simulink model "non_linear_cartesian_controller"  (R2024b)
settings: Solver=VariableStepAuto  StartTime=0.0  StopTime=40  RelTol=1e-3
undefined symbols (not defined in the file or in its folder): extractTop2x2, non_linear_m, non_linear_vcfg
libraries: roblocks x6

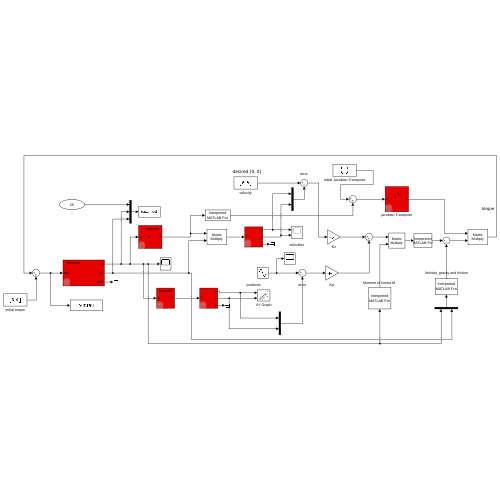
[thumbnail: Simulink's stored preview of the top-level diagram]
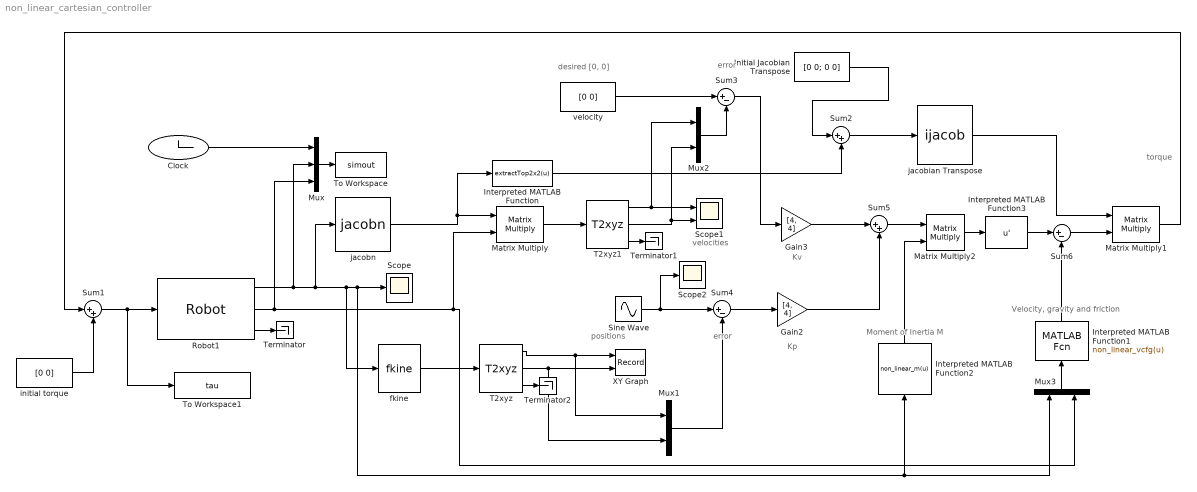
== system non_linear_cartesian_controller ==
  note: Kp
  note: Kv
  note: Moment of Inertia M
  note: error
  note: error
  note: velocities
  note: desired [0, 0]
  note: positions
  note: torque
  note: Velocity, gravity and friction
  Clock : Clock
  Gain2 : Gain  Gain=[4, 4]
  Gain3 : Gain  Gain=[4, 4]
  Initial Jacobian Transpose : Constant  Value=[0 0; 0 0]
  Interpreted MATLAB Function : MATLABFcn  MATLABFcn=extractTop2x2(u)  OutputDimensions=[2 2]  Output1D=off
  Interpreted MATLAB Function1 : MATLABFcn  MATLABFcn=non_linear_vcfg(u)  OutputDimensions=[2 1]  Output1D=off
  Interpreted MATLAB Function2 : MATLABFcn  MATLABFcn=non_linear_m(u)  OutputDimensions=[2 2]  Output1D=off
  Interpreted MATLAB Function3 : MATLABFcn  MATLABFcn=u'  OutputDimensions=[2 1]  Output1D=off
  Matrix Multiply : Product  Multiplication=Matrix(*)
  Matrix Multiply1 : Product  Multiplication=Matrix(*)
  Matrix Multiply2 : Product  Multiplication=Matrix(*)
  Mux : Mux  Inputs=3
  Mux1 : Mux  Inputs=2
  Mux2 : Mux  Inputs=2
  Mux3 : Mux  Inputs=2
  Robot1 : roblocks/Robot  robot=robot  q0=[0 0 0 0 0 0]
      link override Integrator: InitialCondition=[1 1]
      link override Integrator1: InitialCondition=[1 1]
  Scope : Scope
  Scope1 : Scope  NumInputPorts=2
  Scope2 : Scope
  Sine Wave : Sin  Amplitude=0.5  Bias=1  Frequency=1.256  SampleTime=0
  Sum1 : Sum  Inputs=|++
  Sum2 : Sum  Inputs=|++
  Sum3 : Sum  Inputs=|+-
  Sum4 : Sum  Inputs=|+-
  Sum5 : Sum  Inputs=|++
  Sum6 : Sum  Inputs=|+-
  T2xyz : roblocks/T2xyz
  T2xyz1 : roblocks/T2xyz
      link override MATLAB Fcn: MATLABFcn=transljac(u)
  Terminator : Terminator
  Terminator1 : Terminator
  Terminator2 : Terminator
  To Workspace : ToWorkspace  VariableName=simout  SampleTime=-1
  To Workspace1 : ToWorkspace  VariableName=tau  SampleTime=-1
      settings: Save2DSignal=2-D array (concatenate along first dimension)
  XY Graph : Record  FileSettingsInternal="{\"entries\":[{\"content\":{\"excelSettings\":{\"content\":{},\"type\":\"Streamout.ExcelSettings\"}},\"type\":\"Streamout.FileSettingStorage\",\"uuid\":\"\"}],\"packageUris\":[\"http:\\/\\/schema.mathworks.com\\/mf0\\/streamout_blocks\\/R2020a\"],\"version\":\"1.0\"}"  Layout=[1 1]  SignalsInternal="{\"entries\":[{\"content\":{\"signals\":[{\"content\":{\"blockPath\":[],\"dimensions\":[1],\"domain\":\"\",\"lineColor\":\"#a2142f\",\"plots\":[ 1 ],\"port\":1,\"sid\":[\"\"],\"signalID\":1,\"signalName\":\"T2xyz:1\"},\"type\":\"RecordBlkView.Signal\",\"uuid\":\"\"},{\"content\":{\"blockPath\":[],\"dimensions\":[1],\"domain\":\"\",\"lineColor\":\"#139fff\",\"plots\":[ 1 ],\"port\":2,\"sid\":[\"\"],\"signalID\":2,\"signalName\":\"T2xyz:2\"},\"type\":\"RecordBlkView.Signal\",\"uuid\":\"\"}]},\"type\":\"RecordBlkView.InputSignals\",\"uuid\":\"\"}],\"packageUris\":[\"http:\\/\\/schema.mathworks.com\\/mf0\\/streamout_blocks\\/R2020a\"],\"version\":\"1.0\"}"  VisualizationBindings="{\"xyplotplugin\":{\"info\":[{\"series\":[{\"bindingParametersList\":[{\"parameter\":\"X-Axis\",\"signalID\":1,\"signalName\":\"T2xyz:1\"},{\"parameter\":\"Y-Axis\",\"signalID\":2,\"signalName\":\"T2xyz:2\"}],\"seriesID\":0}],\"subplotID\":1}]}}"  CompatibilityTag=XY
  fkine : roblocks/fkine  robot=robot
  initial torque : Constant  Value=[0 0]
  jacobian Transpose : roblocks/ijacob
      link override inverse jacobian: MATLABFcn=u'
  jacobn : roblocks/jacobn  robot=robot
      link override MATLAB Fcn: MATLABFcn=jacobn(robot,u)
  velocity : Constant  Value=[0 0]
  wires:
  Gain3/1 -> Sum5/1
  Robot1/3 -> Terminator/1
  T2xyz/1 -> XY Graph/1, Mux1/1
  Sum4/1 -> Gain2/1
  fkine/1 -> T2xyz/1
  Mux/1 -> To Workspace/1
  Mux2/1 -> Sum3/2
  Clock/1 -> Mux/1
  Interpreted MATLAB Function/1 -> Sum2/2
  T2xyz1/1 -> Scope1/1, Mux2/1
  jacobian Transpose/1 -> Matrix Multiply1/1
  Robot1/2 -> Mux3/2, Matrix Multiply/2, Mux/3
  Sine Wave/1 -> Scope2/1, Sum4/1
  Sum3/1 -> Gain3/1
  Gain2/1 -> Sum5/2
  Robot1/1 -> Mux3/1, Interpreted MATLAB Function2/1, Scope/1, fkine/1, jacobn/1, Mux/2
  T2xyz/2 -> XY Graph/2, Mux1/2
  velocity/1 -> Sum3/1
  jacobn/1 -> Interpreted MATLAB Function/1, Matrix Multiply/1
  Initial Jacobian Transpose/1 -> Sum2/1
  Matrix Multiply/1 -> T2xyz1/1
  T2xyz1/2 -> Scope1/2, Mux2/2
  initial torque/1 -> Sum1/2
  Mux1/1 -> Sum4/2
  Matrix Multiply1/1 -> Sum1/1
  Sum2/1 -> jacobian Transpose/1
  Sum6/1 -> Matrix Multiply1/2
  Interpreted MATLAB Function1/1 -> Sum6/2
  Mux3/1 -> Interpreted MATLAB Function1/1
  Interpreted MATLAB Function2/1 -> Matrix Multiply2/2
  Sum5/1 -> Matrix Multiply2/1
  Interpreted MATLAB Function3/1 -> Sum6/1
  Matrix Multiply2/1 -> Interpreted MATLAB Function3/1
  Sum1/1 -> To Workspace1/1, Robot1/1
  T2xyz1/3 -> Terminator1/1
  T2xyz/3 -> Terminator2/1
